simulink model "Lab7_1"  (R2023a)
settings: Solver=FixedStepAuto  StartTime=0.0  StopTime=3.0  FixedStep=0.0001  RelTol=1e-3
undefined symbols (not defined in the file): A, B, D, G_2, x1
settings Model: Creator=Дети  LastModifiedBy=user

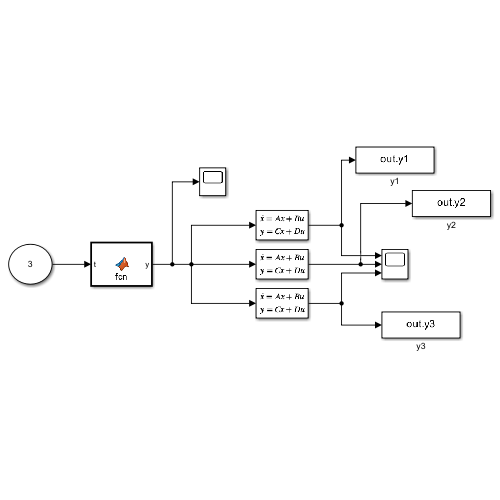
[thumbnail: Simulink's stored preview of the top-level diagram]
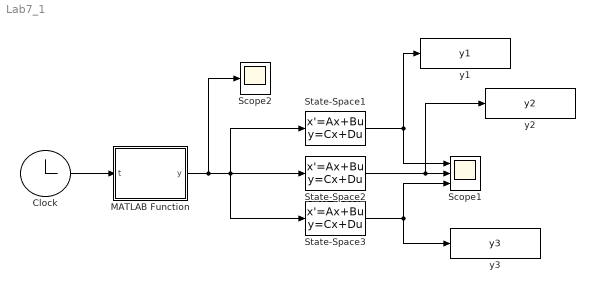
== system Lab7_1 ==
  Clock : Clock
  MATLAB Function : MATLAB Function  TreatAsAtomicUnit=on
  Scope1 : Scope  NumInputPorts=3
  Scope2 : Scope
  State-Space1 : StateSpace  A=[1 2 -1; -6 -7 -2; 6 6 1]  B=B  C=[1 0 0]  D=D  InitialCondition=0
  State-Space2 : StateSpace  A=A  B=B  C=[0 1 0]  D=D  InitialCondition=0
  State-Space3 : StateSpace  A=A  B=B  C=[0 0 1]  D=D  InitialCondition=0
  y1 : ToWorkspace  VariableName=y1  SaveFormat=Timeseries  SampleTime=-1
  y2 : ToWorkspace  VariableName=y2  SaveFormat=Timeseries  SampleTime=-1
  y3 : ToWorkspace  VariableName=y3  SaveFormat=Timeseries  SampleTime=-1
  wires:
  MATLAB Function/1(y) -> Scope2/1, State-Space3/1, State-Space2/1, State-Space1/1
  Clock/1 -> MATLAB Function/1(t)
  State-Space2/1 -> y2/1, Scope1/2
  State-Space3/1 -> Scope1/3, y3/1
  State-Space1/1 -> y1/1, Scope1/1

== matlab function Lab7_1/MATLAB Function ==
  data: t input; y output; A parameter; B parameter; G_2 parameter; x1 parameter
function y = fcn(t, A, B, G_2, x1)
G = [1.0078 -1.4438 0.1155; -1.4438 2.5336 -0.5385;
    0.1155 -0.5385 0.5385];
y = B'*expm(A'*(3-t))*inv(G_2)*x1;
